simulink model "prot_filtro"  (R2016b)
settings: Solver=VariableStepAuto  StartTime=0.0  StopTime=1e-3  RelTol=1e-3
values from neighbouring files (symbols this model uses):
  B = fir1(N, Fc/(Fs/2))    [coef_filtro.m]    (also in sinal_para_vhdl.m = fir1(100, 1e2/(Fs/2)))
  freq = 2500    [coef_filtro.m]
  freq_alta = freq*10    (= 25000)    [coef_filtro.m]
  Ts = 1e-6    (= 1e-06)    [coef_filtro.m]    (also in sinal_para_vhdl.m; untitled2.m = 0.000125)
settings Model: Creator=root  LastModifiedBy=root

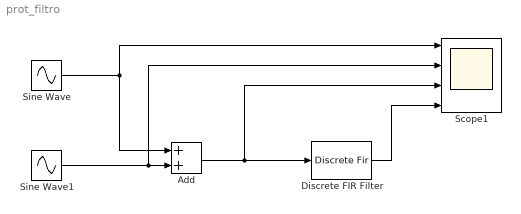
== system prot_filtro ==
  Add : Sum
  Discrete FIR Filter : DiscreteFir  Coefficients=B
  Scope1 : Scope  NumInputPorts=4
  Sine Wave : Sin  Frequency=2*pi*freq  SampleTime=Ts
  Sine Wave1 : Sin  Frequency=2*pi*freq_alta  SampleTime=Ts
  wires:
  Add/1 -> Discrete FIR Filter/1, Scope1/3
  Sine Wave/1 -> Scope1/1, Add/1
  Sine Wave1/1 -> Scope1/2, Add/2
  Discrete FIR Filter/1 -> Scope1/4
